simulink library "InertialAndTargetPointing"  (R2014b)
settings: Solver=VariableStepAuto  StartTime=0.0  StopTime=10.0  RelTol=1e-3
undefined symbols (not defined in the file): ConfParam
libraries: AdvancedMux x2, Normalization x2, AdvancedDemux x1, ComputeNorm3D x1, InertialPointing x1, ScalarProduct3D x1, TargetPointing x1
settings Model: Creator=y.akisheva  LastModifiedBy=Hp
settings DataIOCC: SaveFormat=Dataset
settings OptimizationCC: UseDivisionForNetSlopeComputation=off  SimCompilerOptimization=off
settings DebuggingCC: SolverPrmCheckMsg=none  FrameProcessingCompatibilityMsg=error  AllowSymbolicDim=off
settings HardwareCC: ProdBitPerPointer=64  ProdLargestAtomicFloat=Float  ProdIntDivRoundTo=Zero  ProdEndianess=LittleEndian  ProdWordSize=64  ProdHWDeviceType=Intel->x86-64 (Windows64)
settings RTWCC: RTWCompilerOptimization=off
settings GRTTargetCC: GeneratePreprocessorConditionals=Use local settings
settings ConfigComp: CovMetricSettings=dw  CovHtmlReporting=on  CovSaveCumulativeToWorkspaceVar=on  CovSaveSingleToWorkspaceVar=on  CovExternalEMLEnable=off

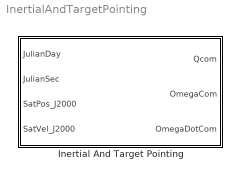
== system InertialAndTargetPointing ==
  "Inertial And Target Pointing " : Subsystem

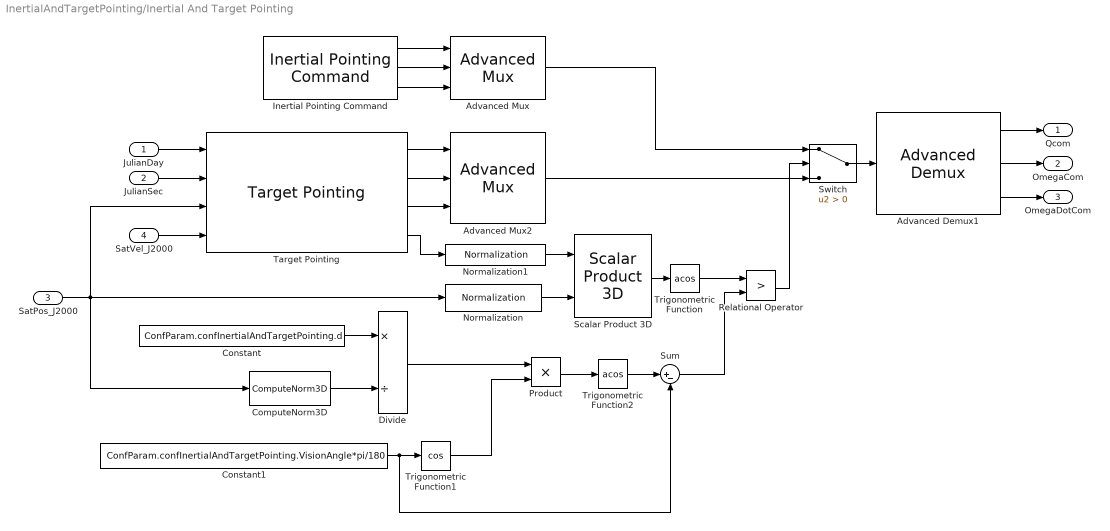
== system InertialAndTargetPointing/Inertial And Target Pointing  ==
  JulianDay : Inport
  JulianSec : Inport  Port=2
  SatPos_J2000 : Inport  Port=3
  SatVel_J2000 : Inport  Port=4
  Advanced Demux1 : AdvancedDemux/Advanced Demux
  Advanced Mux : AdvancedMux/Advanced Mux
  Advanced Mux2 : AdvancedMux/Advanced Mux
  ComputeNorm3D : ComputeNorm3D/ComputeNorm3D
  Constant : Constant  Value=ConfParam.confInertialAndTargetPointing.d
  Constant1 : Constant  Value=ConfParam.confInertialAndTargetPointing.VisionAngle*pi/180
  Divide : Product  Inputs=*/
  Inertial Pointing Command : InertialPointing/Inertial Pointing Command
  Normalization : Normalization/Normalization
  Normalization1 : Normalization/Normalization
  Product : Product
  Relational Operator : RelationalOperator  Operator=>  OutDataTypeStr=boolean
  Scalar Product 3D : ScalarProduct3D/Scalar Product 3D
  Sum : Sum  Inputs=|+-
  Switch : Switch  Criteria=u2 > Threshold
  Target Pointing : TargetPointing/Target Pointing
  Trigonometric Function : Trigonometry  Operator=acos
  Trigonometric Function1 : Trigonometry  Operator=cos
  Trigonometric Function2 : Trigonometry  Operator=acos
  Qcom : Outport
  OmegaCom : Outport  Port=2
  OmegaDotCom : Outport  Port=3
  wires:
  SatVel_J2000/1 -> Target Pointing/4
  JulianSec/1 -> Target Pointing/2
  JulianDay/1 -> Target Pointing/1
  Target Pointing/4 -> Normalization1/1
  Scalar Product 3D/1 -> Trigonometric Function/1
  Trigonometric Function/1 -> Relational Operator/1
  Normalization/1 -> Scalar Product 3D/2
  Normalization1/1 -> Scalar Product 3D/1
  Advanced Demux1/3 -> OmegaDotCom/1
  Advanced Demux1/2 -> OmegaCom/1
  Advanced Demux1/1 -> Qcom/1
  Inertial Pointing Command/1 -> Advanced Mux/1
  Target Pointing/3 -> Advanced Mux2/3
  Inertial Pointing Command/3 -> Advanced Mux/3
  Target Pointing/2 -> Advanced Mux2/2
  Inertial Pointing Command/2 -> Advanced Mux/2
  Target Pointing/1 -> Advanced Mux2/1
  Switch/1 -> Advanced Demux1/1
  Advanced Mux/1 -> Switch/1
  Advanced Mux2/1 -> Switch/3
  SatPos_J2000/1 -> ComputeNorm3D/1, Normalization/1, Target Pointing/3
  Constant/1 -> Divide/1
  ComputeNorm3D/1 -> Divide/2
  Divide/1 -> Product/1
  Trigonometric Function1/1 -> Product/2
  Product/1 -> Trigonometric Function2/1
  Trigonometric Function2/1 -> Sum/1
  Constant1/1 -> Sum/2, Trigonometric Function1/1
  Sum/1 -> Relational Operator/2
  Relational Operator/1 -> Switch/2
